simulink model "temp2"  (Simulink 7.7)
settings: Solver=ode45  StartTime=0.0  StopTime=20.0  RelTol=1e-3
PreLoadFcn:
  | EbNo = 16; Errors = 188; Bits = 1e8; M = 256; N = 64; Ts = (1/22050); constellation; InnerInterleaverBitTable
undefined symbols (not defined in the file or in its folder): figposition, Fs, get, rsgenpoly, sided, Two
libraries: commblkintrlv2 x6, commutil2 x4, commsink2 x3, commblkcod2 x2, dspsnks4 x2, commdigbbndam3 x2, commcnvcod2 x2, dspsigops x2, dspxfrm3 x2, commcnvintrlv2 x2, dspsrcs4 x1
settings Model: Creator=katsikas  LastModifiedBy=katsikas

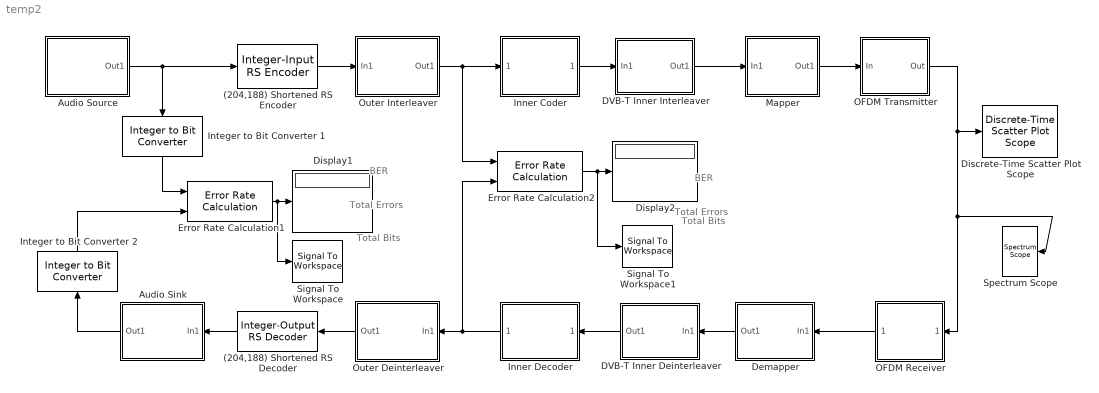
== system temp2 ==
  note: BER
  note: Total Errors
  note: Total Bits
  note: BER
  note: Total Bits
  note: Total Errors
  (204,188) Shortened RS Decoder : commblkcod2/Integer-Output RS Decoder  n=204  k=188  specPrimPoly=off  prPoly=[1 0 1 1]  specGenPoly=off  genPoly=rsgenpoly(7,3)  specPuncture=off  punctVec=[ones(2,1); zeros(2,1)]  specErasurePort=off  showNumErr=off
  (204,188) Shortened RS Encoder : commblkcod2/Integer-Input RS Encoder  n=204  k=188  specPrimPoly=off  prPoly=[1 0 1 1]  specGenPoly=off  genPoly=rsgenpoly(7,3)  specPuncture=off  punctVec=[ones(2,1); zeros(2,1)]
  Audio Sink : Subsystem
  Audio Source : Subsystem
  DVB-T Inner Deinterleaver : Subsystem  mask(DVB-T Inner Deinterleaver){}
      mask init:
      | fullILVec = [(1:126) ...
      |  (rem([0:125]+63,126) +1 + 126     ) ...
      |  (rem([0:125]+105,126)+1 + (2*126) ) ...
      |  (rem([0:125]+42,126) +1 + (3*126) ) ...
      |  (rem([0:125]+21,126) +1 + (4*126) ) ...
      |  (rem([0:125]+84,126) +1 + (5*126) )];
      mask Display: disp('DVB-T\nInner\nDeinterleaver')
  DVB-T Inner Interleaver : Subsystem  mask(DVB-T Inner Interleaver){}
      mask init: same as temp2/DVB-T Inner Deinterleaver
      mask Display: disp('DVB-T\nInner\nInterleaver')
  Demapper : Subsystem
      mask Type: DVB-T 64-QAM Demapper
      mask Display: disp('DVB-T\n64-QAM\nDemapper')
  Discrete-Time Scatter Plot Scope : commsink2/Discrete-Time Scatter Plot Scope  Tag=ScatterPlot  SystemSampleTime=-1  sampPerSymb=1  offsetEye=0  numTraces=40  numNewFrames=40  LineMarkers=.  LineColors=b  fading=on  render=on  AxisGrid=on  xMin=-0.0409978671890575  xMax=0.0505226367467033  yMin=-0.0477741534548735  yMax=0.0437463504808873  inphaseLabel=In-phase Amplitude  quadratureLabel=Quadrature Amplitude  openScopeAtSimStart=on  FrameNumber=off  FigPos=get(0,'defaultfigureposition');  figTitle=Scatter Plot  numLinesMax=8  block_type_=scatter
  Display1 : Display
  Display2 : Display
  Error Rate Calculation1 : commsink2/Error Rate Calculation  N=188*17*8  st_delay=0  cp_mode=Entire frame  subframe=[]  PMode=Port  WsName=e2  RsMode2=off  stop=off  numErr=Errors  maxBits=Bits
  Error Rate Calculation2 : commsink2/Error Rate Calculation  N=1632*6  st_delay=0  cp_mode=Entire frame  subframe=[]  PMode=Port  WsName=e1  RsMode2=off  stop=off  numErr=100  maxBits=1e6
  Inner Coder : Subsystem
      mask Display: disp('Rate 3/4\nPunctured\nConvolutional\nCode');
  Inner Decoder : Subsystem
      mask Display: disp('Viterbi\nDecoder')
  Integer to Bit Converter 1 : commutil2/Integer to Bit Converter  nbits=8  signedInputValues=Unsigned  bitOrder=MSB first  outDtype=boolean
  Integer to Bit Converter 2 : commutil2/Integer to Bit Converter  nbits=8  signedInputValues=Unsigned  bitOrder=MSB first  outDtype=boolean
  Mapper : Subsystem
      mask Type: DVB-T 64-QAM Mapper
      mask Display: disp('DVB-T\n64-QAM\nMapper')
  OFDM Receiver : Subsystem
      mask Display: disp('OFDM\nReceiver')
  OFDM Transmitter : Subsystem
      mask Display: disp('OFDM\nTransmitter')
  Outer Deinterleaver : Subsystem
      mask Display: disp('Convolutional\nDeinterleaver\nI=12')
  Outer Interleaver : Subsystem
      mask Display: disp('Convolutional\nInterleaver\nI=12')
  Signal To Workspace : SignalToWorkspace  VariableName=BER  SaveFormat=Array  Save2DMode=2-D array (concatenate along first dimension)
      settings: CopyFcn=dspblkcopystw(gcbh);  MaxDataPoints=1
  Signal To Workspace1 : SignalToWorkspace  VariableName=BER1  SaveFormat=Array  Save2DMode=2-D array (concatenate along first dimension)
      settings: CopyFcn=dspblkcopystw(gcbh);  MaxDataPoints=1
  Spectrum Scope : dspsnks4/Spectrum Scope  SystemSampleTime=-1  ScopeProperties=off  Domain=Frequency  HorizSpan=1  UseBuffer=off  BufferSize=128  Overlap=64  TreatMby1Signals=One channel  inpFftLenInherit=off  FFTlength=128  numAvg=2  DisplayProperties=on  AxisGrid=on  Memory=off  FrameNumber=off  AxisLegend=off  AxisZoom=off  OpenScopeAtSimStart=on  OpenScopeImmediately=off  FigPos=figposition([1 7 36 45])  AxisProperties=off  XUnits=Hertz  XRange=Two-sided ((-Fs/2...Fs/2])  XDisplay=0  InheritXIncr=on  XIncr=1.0  XLabel=Samples  XLimit=Auto  YUnits=dBW/Hertz  XMax=1  XMin=0  YLabel=Power spectral density, dBW/Hz  LineProperties=off  wintypeSpecScope=Hann  RsSpecScope=50  betaSpecScope=5  winsampSpecScope=Periodic  XAxisParamsVer=6.9  isFrameUpgraded=on
      settings: YMin=-140  YMax=-90
  wires:
  Audio Source/1(Out1) -> Integer to Bit Converter 1/1, (204,188) Shortened RS Encoder/1
  (204,188) Shortened RS Encoder/1 -> Outer Interleaver/1(In1)
  Outer Deinterleaver/1(Out1) -> (204,188) Shortened RS Decoder/1
  Error Rate Calculation1/1 -> Display1/1, Signal To Workspace/1
  Integer to Bit Converter 2/1 -> Error Rate Calculation1/2
  Integer to Bit Converter 1/1 -> Error Rate Calculation1/1
  (204,188) Shortened RS Decoder/1 -> Audio Sink/1(In1)
  Outer Interleaver/1(Out1) -> Error Rate Calculation2/1, Inner Coder/1(Uncoded symbols)
  OFDM Transmitter/1(Out) -> Discrete-Time Scatter Plot Scope/1, OFDM Receiver/1(Received signal), Spectrum Scope/1
  OFDM Receiver/1(OFDM Spectrum) -> Demapper/1(In1)
  DVB-T Inner Deinterleaver/1(Out1) -> Inner Decoder/1(Received bits)
  Inner Decoder/1(Decoded symbols) -> Outer Deinterleaver/1(In1), Error Rate Calculation2/2
  Demapper/1(Out1) -> DVB-T Inner Deinterleaver/1(In1)
  Mapper/1(Out1) -> OFDM Transmitter/1(In)
  Error Rate Calculation2/1 -> Display2/1, Signal To Workspace1/1
  DVB-T Inner Interleaver/1(Out1) -> Mapper/1(In1)
  Inner Coder/1(Coded bits) -> DVB-T Inner Interleaver/1(In1)
  Audio Sink/1(Out1) -> Integer to Bit Converter 2/1

== system temp2/Audio Sink ==
  In1 : Inport
  Received Scope : dspsnks4/Time Scope
  Out1 : Outport
  wires:
  In1/1 -> Received Scope/1, Out1/1

== system temp2/Audio Source ==
  From Multimedia File : dspsrcs4/From Multimedia File  inputFilename=speech_dft.avi  loop=on  numPlays=inf  outputStreams=Audio only  videoDataType=single  audioDataType=uint8  inheritSampleTime=on  userDefinedSampleTime=Ts  noAudioOutput=off  isIntensityVideo=off  fourcc=RGB  colorVideoFormat=Separate color signals  outputEOF=off  dataOrg=Column-major  audioFrameSize=188  computeAudioFrameSize=off
  Out1 : Outport
  wires:
  From Multimedia File/1 -> Out1/1

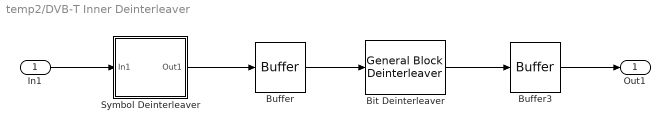
== system temp2/DVB-T Inner Deinterleaver ==
  In1 : Inport
  Bit Deinterleaver : commblkintrlv2/General Block Deinterleaver  elements=BitInterleaverTable
  Buffer : Buffer  N=756  TreatMby1Signals=One channel
  Buffer3 : Buffer  N=2176  TreatMby1Signals=One channel
  Symbol Deinterleaver : Subsystem
      mask Display:
      | port_label('input', 1, '')
      | port_label('output', 1, '')
      | disp('Symbol\nDeinterleaver')
  Out1 : Outport
  wires:
  Buffer/1 -> Bit Deinterleaver/1
  In1/1 -> Symbol Deinterleaver/1(In1)
  Bit Deinterleaver/1 -> Buffer3/1
  Buffer3/1 -> Out1/1
  Symbol Deinterleaver/1(Out1) -> Buffer/1

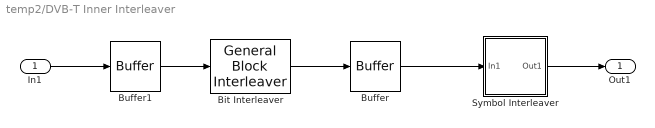
== system temp2/DVB-T Inner Interleaver ==
  In1 : Inport
  Bit Interleaver : commblkintrlv2/General Block Interleaver  elements=BitInterleaverTable
  Buffer : Buffer  N=9072  TreatMby1Signals=One channel
  Buffer1 : Buffer  N=756  TreatMby1Signals=One channel
  Symbol Interleaver : Subsystem
      mask Display:
      | port_label('input', 1, '')
      | port_label('output', 1, '')
      | disp('Symbol\nInterleaver')
  Out1 : Outport
  wires:
  Buffer1/1 -> Bit Interleaver/1
  In1/1 -> Buffer1/1
  Bit Interleaver/1 -> Buffer/1
  Symbol Interleaver/1(Out1) -> Out1/1
  Buffer/1 -> Symbol Interleaver/1(In1)

== system temp2/Demapper ==
  In1 : Inport
  Demodulator : commdigbbndam3/Rectangular QAM Demodulator Baseband  M=N  PowType=Average Power  MinDist=2  AvgPow=1  PeakPow=1  Ph=0  Dec=User-defined  Mapping=map_constellation  OutType=Bit  DecType=Hard decision  VarSource=Port  Variance=0.03  outDtype1=double  outDtype2=double  derotateFactorWordLen=16  denormFactorWordLen=16  prodOutWordLen=32  prodOutRoundingMode=Floor  prodOutOverflowMode=Wrap  sumWordLen=32
  Out1 : Outport
  wires:
  In1/1 -> Demodulator/1
  Demodulator/1 -> Out1/1

== system temp2/Inner Coder ==
  Uncoded symbols : Inport
  Convolutional  Encoder : commcnvcod2/Convolutional Encoder  trellis=poly2trellis(7, [171 133])  opMode=Continuous  DelayedResetAction=off  hasIniStPort=off  hasFinStPort=off  usePuncVector=on  punctureVector=[1 1 0 1 1 0]'  reset=Unused parameter value
  Coded bits : Outport
  wires:
  Convolutional  Encoder/1 -> Coded bits/1
  Uncoded symbols/1 -> Convolutional  Encoder/1

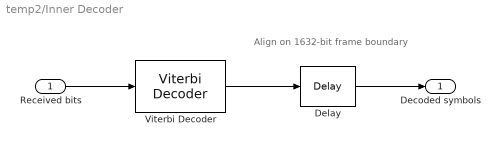
== system temp2/Inner Decoder ==
  note: Align on 1632-bit
      | frame boundary
  Received bits : Inport
  Delay : dspsigops/Delay  InputProcessing=Columns as channels (frame based)  dly_unit=Samples  delay=584+69  ic_detail=off  dif_ic_for_ch=off  dif_ic_for_dly=off  ic=0  reset_popup=None
  Viterbi Decoder : commcnvcod2/Viterbi Decoder  trellis=poly2trellis(7, [171 133])  isPunctured=on  punctureVector=[1 1 0 1 1 0]'  erasures=off  dectype=Hard decision  runSigValErrCheck=off  nsdecb=4  smWordLength=16  tbdepth=136  opmode=Continuous  reset=off  outDataType=boolean
  Decoded symbols : Outport
  wires:
  Viterbi Decoder/1 -> Delay/1
  Received bits/1 -> Viterbi Decoder/1
  Delay/1 -> Decoded symbols/1

== system temp2/Mapper ==
  In1 : Inport
  Modulator : commdigbbndam3/Rectangular QAM Modulator Baseband  M=N  InType=Bit  Enc=User-defined  Mapping=map_constellation  PowType=Average Power  MinDist=2  AvgPow=1  PeakPow=1  Ph=0  outDtype=double  outWordLen=16  outUDDataType=sfix(16)  outFracLenMode=Best precision  outFracLen=15
  Out1 : Outport
  wires:
  In1/1 -> Modulator/1
  Modulator/1 -> Out1/1

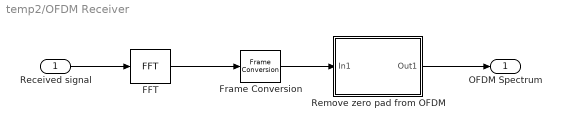
== system temp2/OFDM Receiver ==
  Received signal : Inport
  FFT : dspxfrm3/FFT  CompMethod=Table lookup  TableOpt=NEW  TableOptActive=Speed  BitRevOrder=off  InheritFFTLength=on  FFTLength=64  RowConvenienceOn=on  SkipNorm=off  firstCoeffMode=Specify word length  firstCoeffWordLength=16  firstCoeffFracLength=15  firstCoeffDataTypeStr=fixdt(1,16)  firstCoeffLastDataTypeStr=fixdt(1,16)  outputMin=[]  outputMax=[]  accumDataTypeStr=Inherit: Same as product output  accumLastDataTypeStr=Inherit: Same as product output  roundingMode=Floor  overflowMode=off
  Frame Conversion : FrameConversion
  Remove zero pad from OFDM : Subsystem
      mask Display: disp('Remove zero\npad from OFDM');
  OFDM Spectrum : Outport
  wires:
  Remove zero pad from OFDM/1(Out1) -> OFDM Spectrum/1
  Received signal/1 -> FFT/1
  FFT/1 -> Frame Conversion/1
  Frame Conversion/1 -> Remove zero pad from OFDM/1(In1)

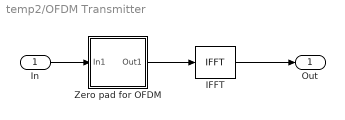
== system temp2/OFDM Transmitter ==
  In : Inport
  IFFT : dspxfrm3/IFFT  CompMethod=Table lookup  TableOpt=HYBRID  TableOptActive=Speed  BitRevOrder=off  cs_in=off  SkipNorm=on  InheritFFTLength=on  FFTLength=64  mode=Complex  outSamplingMode=Frame based  RowConvenienceOn=on  firstCoeffMode=Specify word length  firstCoeffWordLength=16  firstCoeffFracLength=15  firstCoeffDataTypeStr=fixdt(1,16)  firstCoeffLastDataTypeStr=fixdt(1,16)  outputMin=[]  outputMax=[]  accumDataTypeStr=Inherit: Same as product output  accumLastDataTypeStr=Inherit: Same as product output  roundingMode=Floor  overflowMode=off
  Zero pad for OFDM : Subsystem
      mask Display: disp('Zero pad\nfor OFDM');
  Out : Outport
  wires:
  IFFT/1 -> Out/1
  In/1 -> Zero pad for OFDM/1(In1)
  Zero pad for OFDM/1(Out1) -> IFFT/1

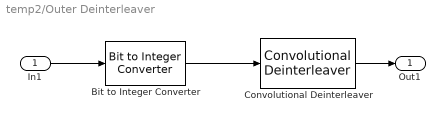
== system temp2/Outer Deinterleaver ==
  In1 : Inport
  Bit to Integer Converter : commutil2/Bit to Integer Converter  nbits=8  bitOrder=MSB first  signedOutputValues=Unsigned  outDtype=uint8  outDtypeSigned=Inherit via internal rule
  Convolutional Deinterleaver : commcnvintrlv2/Convolutional Deinterleaver  SystemSampleTime=-1  N=12  B=17  ic=0
  Out1 : Outport
  wires:
  In1/1 -> Bit to Integer Converter/1
  Convolutional Deinterleaver/1 -> Out1/1
  Bit to Integer Converter/1 -> Convolutional Deinterleaver/1

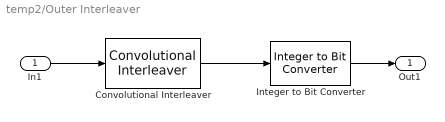
== system temp2/Outer Interleaver ==
  In1 : Inport
  Convolutional Interleaver : commcnvintrlv2/Convolutional Interleaver  SystemSampleTime=-1  N=12  B=17  ic=0
  Integer to Bit Converter : commutil2/Integer to Bit Converter  nbits=8  signedInputValues=Unsigned  bitOrder=MSB first  outDtype=boolean
  Out1 : Outport
  wires:
  Integer to Bit Converter/1 -> Out1/1
  Convolutional Interleaver/1 -> Integer to Bit Converter/1
  In1/1 -> Convolutional Interleaver/1

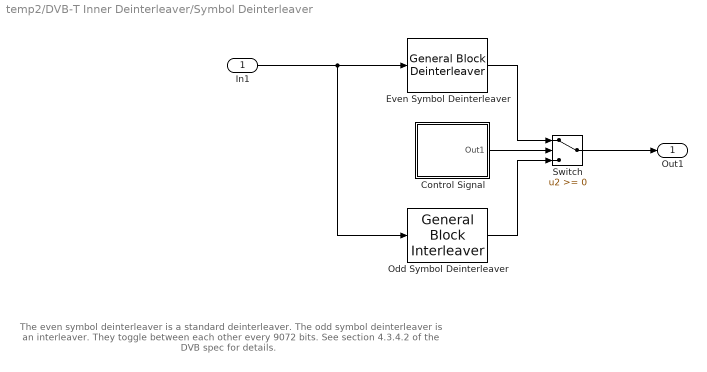
== system temp2/DVB-T Inner Deinterleaver/Symbol Deinterleaver ==
  note: The even symbol deinterleaver is a standard deinterleaver.  The odd symbol deinterleaver is an interleaver.  They toggle
      | between each other every 9072 bits.  See section 4.3.4.2 of the DVB spec for details.
  In1 : Inport
  Control Signal : Subsystem
      mask Display:
      | port_label('output', 1, 'ctrl')
      | disp('Control\nSignal')
  Even Symbol Deinterleaver : commblkintrlv2/General Block Deinterleaver  elements=SymbolInterleaverTable
  Odd Symbol Deinterleaver : commblkintrlv2/General Block Interleaver  elements=SymbolInterleaverTable
  Switch : Switch
  Out1 : Outport
  wires:
  In1/1 -> Odd Symbol Deinterleaver/1, Even Symbol Deinterleaver/1
  Switch/1 -> Out1/1
  Control Signal/1(Out1) -> Switch/2
  Even Symbol Deinterleaver/1 -> Switch/1
  Odd Symbol Deinterleaver/1 -> Switch/3

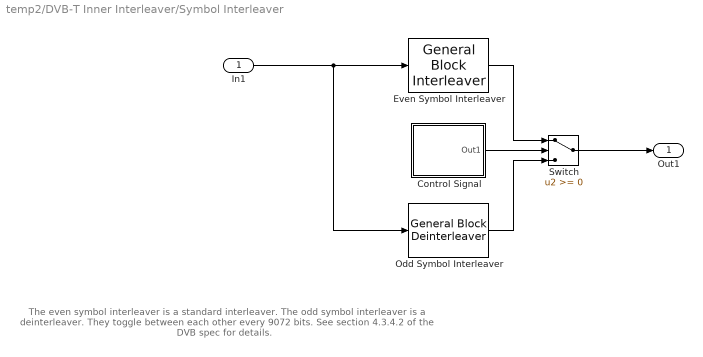
== system temp2/DVB-T Inner Interleaver/Symbol Interleaver ==
  note: The even symbol interleaver is a standard interleaver.  The odd symbol interleaver is a deinterleaver.  They toggle
      | between each other every 9072 bits.  See section 4.3.4.2 of the DVB spec for details.
  In1 : Inport
  Control Signal : Subsystem
      mask Display:
      | port_label('output', 1, 'ctrl')
      | disp('Control\nSignal')
  Even Symbol Interleaver : commblkintrlv2/General Block Interleaver  elements=SymbolInterleaverTable
  Odd Symbol Interleaver : commblkintrlv2/General Block Deinterleaver  elements=SymbolInterleaverTable
  Switch : Switch
  Out1 : Outport
  wires:
  In1/1 -> Even Symbol Interleaver/1, Odd Symbol Interleaver/1
  Switch/1 -> Out1/1
  Control Signal/1(Out1) -> Switch/2
  Even Symbol Interleaver/1 -> Switch/1
  Odd Symbol Interleaver/1 -> Switch/3

== system temp2/OFDM Receiver/Remove zero pad from OFDM ==
  In1 : Inport
  Selector : Selector  NumberOfDimensions=2  InputPortWidth=2048  IndexOptions=Index vector (dialog),Select all  Indices=[1:756 1293:2048],1  OutputSizes=1,1
  Out1 : Outport
  wires:
  In1/1 -> Selector/1
  Selector/1 -> Out1/1

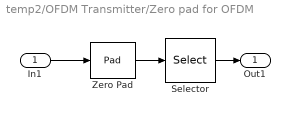
== system temp2/OFDM Transmitter/Zero pad for OFDM ==
  In1 : Inport
  Selector : Selector  NumberOfDimensions=2  InputPortWidth=2048  IndexOptions=Index vector (dialog),Select all  Indices="[1:756 1513:2048  757:1512],1"  OutputSizes=1,1
  Zero Pad : dspsigops/Pad  padAlong=Columns  dimsToPad=1  valSrc=Specify via dialog  padVal=0  spec=Output size  padNumOutRowsSpecMethod=User-specified  numOutRows=2048  padNumOutColsSpecMethod=User-specified  numOutCols=1  isVarDimsMode=off  padBeginning=0  padEnd=0  outSizeMode=User-specified  outSize=1  padSigAt=End  trunc_flag=None  roundingMode=Floor  overflowMode=off  truncOrWrapMode=Truncate  wrap_flag=None
  Out1 : Outport
  wires:
  In1/1 -> Zero Pad/1
  Selector/1 -> Out1/1
  Zero Pad/1 -> Selector/1

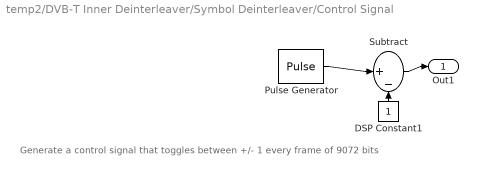
== system temp2/DVB-T Inner Deinterleaver/Symbol Deinterleaver/Control Signal ==
  note: Generate a control signal that toggles between +/- 1 every frame of 9072 bits
  DSP Constant1 : Constant  VectorParams1D=off
  Pulse Generator : DiscretePulseGenerator  Amplitude=2  SampleTime=-1
  Subtract : Sum  Inputs=|+-
  Out1 : Outport
  wires:
  Subtract/1 -> Out1/1
  DSP Constant1/1 -> Subtract/2
  Pulse Generator/1 -> Subtract/1

== system temp2/DVB-T Inner Interleaver/Symbol Interleaver/Control Signal ==
  note: Generate a control signal that toggles between +/- 1 every frame of 9072 bits
  DSP Constant1 : Constant  VectorParams1D=off
  Pulse Generator : DiscretePulseGenerator  Amplitude=2  SampleTime=-1
  Subtract : Sum  Inputs=|+-
  Out1 : Outport
  wires:
  Subtract/1 -> Out1/1
  DSP Constant1/1 -> Subtract/2
  Pulse Generator/1 -> Subtract/1
